simulink subsystem "Leds"  (R2024b)
settings: Solver=VariableStepAuto  StartTime=0.0  StopTime=10.0  RelTol=1e-3
libraries: simulink x2, arduinolib x2
settings Model: Creator=Chenfu  LastModifiedBy=Chenfu
settings OptimizationCC: ReuseModelBlockBuffer=off
settings RTWCC: GPUComputeCapability=3.5

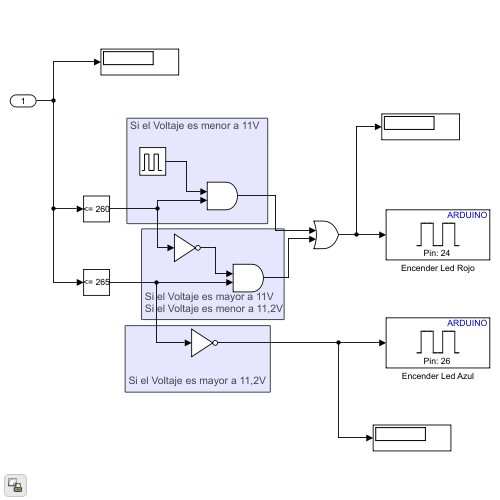
[thumbnail: Simulink's stored preview of the top-level diagram]
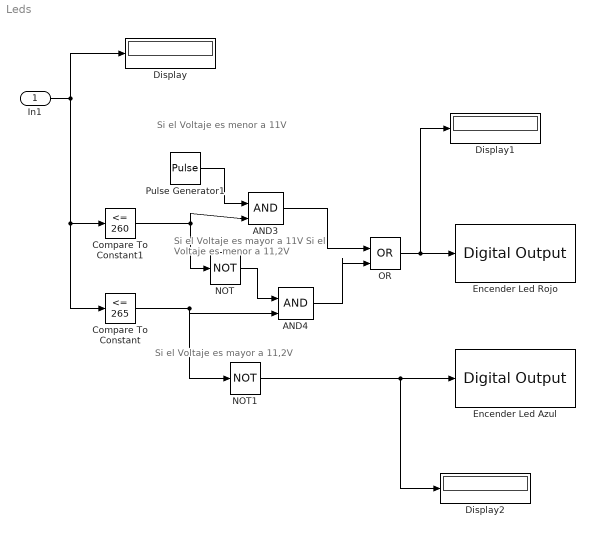
== system Leds ==
  note: Si el Voltaje es mayor a 11,2V
  note: Si el Voltaje es mayor a 11V
      | Si el Voltaje es menor a 11,2V
  note: Si el Voltaje es menor a 11V
  In1 : Inport
  AND3 : Logic  IconShape=distinctive  AllPortsSameDT=off  OutDataTypeStr=boolean
  AND4 : Logic  IconShape=distinctive  AllPortsSameDT=off  OutDataTypeStr=boolean
  Compare To Constant : simulink/Logic and Bit Operations/Compare To Constant  relop=<=  const=265  OutDataTypeStr=boolean
  Compare To Constant1 : simulink/Logic and Bit Operations/Compare To Constant  relop=<=  const=260  OutDataTypeStr=boolean
  Display : Display
  Display1 : Display
  Display2 : Display
  Encender Led Azul : arduinolib/Digital Output  pinNumber=26  Direction=output  blockPlatform=arduino
  Encender Led Rojo : arduinolib/Digital Output  pinNumber=24  Direction=output  blockPlatform=arduino
  NOT : Logic  Operator=NOT  IconShape=distinctive  AllPortsSameDT=off  OutDataTypeStr=boolean
  NOT1 : Logic  Operator=NOT  IconShape=distinctive  AllPortsSameDT=off  OutDataTypeStr=boolean
  OR : Logic  Operator=OR  IconShape=distinctive  AllPortsSameDT=off  OutDataTypeStr=boolean
  Pulse Generator1 : DiscretePulseGenerator  PulseType=Time based  Period=10  PulseWidth=50
  wires:
  Pulse Generator1/1 -> AND3/1
  Compare To Constant1/1 -> NOT/1, AND3/2
  Compare To Constant/1 -> AND4/2, NOT1/1
  NOT/1 -> AND4/1
  OR/1 -> Encender Led Rojo/1, Display1/1
  AND4/1 -> OR/2
  AND3/1 -> OR/1
  NOT1/1 -> Encender Led Azul/1, Display2/1
  In1/1 -> Display/1, Compare To Constant1/1, Compare To Constant/1
